simulink subsystem "MyModel"  (R2023a)
settings: Solver=VariableStepAuto  StartTime=0.0  StopTime=10.0  RelTol=1e-3
settings Model: Creator=KozlovM  LastModifiedBy=agalimov

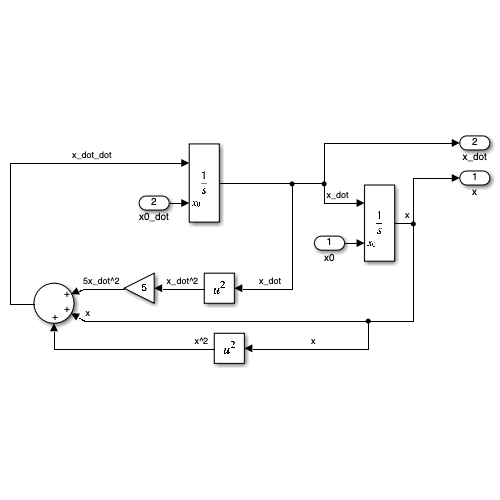
[thumbnail: Simulink's stored preview of the top-level diagram]
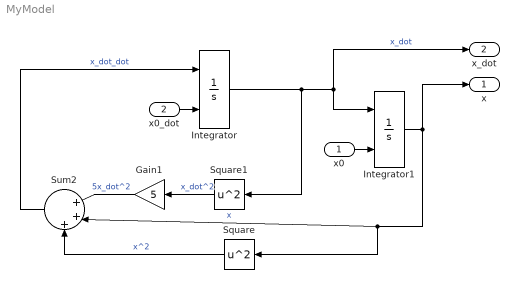
== system MyModel ==
  x0 : Inport
  x0_dot : Inport  Port=2
  Gain1 : Gain  Gain=5
  Integrator : Integrator  InitialConditionSource=external
  Integrator1 : Integrator  InitialConditionSource=external
  Square : Math  Operator=square
  Square1 : Math  Operator=square
  Sum2 : Sum  Inputs=|+++
  x : Outport
  x_dot : Outport  Port=2
  wires:
  Integrator1/1 -> x/1, Sum2/2, Square/1  "x"
  Integrator/1 -> Square1/1, Integrator1/1, x_dot/1  "x_dot"
  x0_dot/1 -> Integrator/2
  x0/1 -> Integrator1/2
  Sum2/1 -> Integrator/1  "x_dot_dot"
  Square/1 -> Sum2/3  "x^2"
  Gain1/1 -> Sum2/1  "5x_dot^2"
  Square1/1 -> Gain1/1  "x_dot^2"
